simulink model "bluetoothzumotest_runMotors"  (R2014a)
settings: Solver=ode3  SolverMode=SingleTasking  StartTime=0.0  StopTime=inf  RelTol=1e-3
libraries: simulink x1, arduinolib x1, ZumoBotLib x1
settings Model: ExtModeTrigDuration=2  Creator=nrattner  LastModifiedBy=sandip
settings OptimizationCC: OptimizeModelRefInitCode=on  LifeSpan=1
settings DebuggingCC: UnderspecifiedInitializationDetection=Classic  SolverPrmCheckMsg=none
settings HardwareCC: ProdBitPerInt=16  ProdBitPerPointer=8  ProdIntDivRoundTo=Zero  ProdEndianess=LittleEndian  ProdWordSize=8  ProdHWDeviceType=Atmel->AVR
settings RTWCC: SystemTargetFile=realtime.tlc  GenerateMakefile=off  TemplateMakefile=realtime.tmf  Description=Run on Target Hardware  RTWVerbose=off  ProcessScript=realtime_make_rtw_hook
settings STFCustomTargetCC: TargetLibSuffix=.a  GenerateSampleERTMain=on  ConcurrentExecutionCompliant=off  GeneratePreprocessorConditionals=Use local settings  ERTCustomFileBanners=on  SupportNonInlinedSFcns=off  SupportVariableSizeSignals=on  MATLABClassNameForMDSCustomization=Simulink.SoftwareTarget.ERTCustomization  GRTInterface=off  SystemTargetFile=realtime.tlc
settings ERTTargetCC: CombineOutputUpdateFcns=off  SupportContinuousTime=on  SupportVariableSizeSignals=on  ExtModeTransport=3  ExtModeMexFile=ext_serial_win32_comm  ExtModeMexArgs=0 1 9600  ERTSrcFileBannerTemplate=realtime_code_template.cgt  ERTHdrFileBannerTemplate=realtime_code_template.cgt  ERTDataSrcFileTemplate=realtime_code_template.cgt  ERTDataHdrFileTemplate=realtime_code_template.cgt  ERTCustomFileTemplate=realtime_file_process.tlc

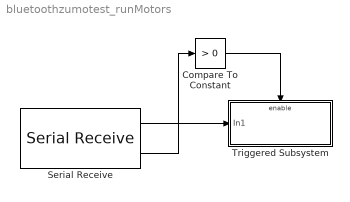
== system bluetoothzumotest_runMotors ==
  Compare To Constant : simulink/Logic and Bit Operations/Compare To Constant  relop=>  const=0  OutDataTypeStr=boolean
  Serial Receive : arduinolib/Serial Receive  portNumber=0  showOutStatus=on  sampleTime=1e-3
  Triggered Subsystem : Subsystem  TreatAsAtomicUnit=on
  wires:
  Serial Receive/1 -> Triggered Subsystem/1(In1)
  Compare To Constant/1 -> Triggered Subsystem/Enable
  Serial Receive/2 -> Compare To Constant/1

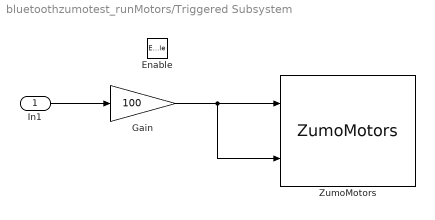
== system bluetoothzumotest_runMotors/Triggered Subsystem ==
  In1 : Inport
  Enable : EnablePort
  Gain : Gain  Gain=100
  ZumoMotors : ZumoBotLib/ZumoMotors  flipLeft=off  flipRight=off
  wires:
  In1/1 -> Gain/1
  Gain/1 -> ZumoMotors/2, ZumoMotors/1
